simulink library "modbus_lib"  (Simulink 7.8)
settings: Solver=ode45  StartTime=0.0  StopTime=10.0  RelTol=1e-3
values from neighbouring files (symbols this model uses):
  relay_sets = xlsread('relay_settings_10272015.xlsx')    [relays_settings_init.m]
  Ts = 80e-6    (= 8e-05)    [global_parameters.m]    (also in scopeBuffer.m)
undefined symbols (not defined in the file or in its folder): angle_threshold, dF_threshold, DiscIntNeverNeededParam, dV_threshold, IOC, TOC, V, VRMSLL
libraries: simulink x24, powerlib_extras x20, powerlib x14, modbus_lib x6, simulink_extras x5, lib_Timer_Counter x4, rtio_generic_modbus x3, dspsigops x2
(part 2 of 2)

== system modbus_lib/CS Modified PLL/Controller ==
  note: Pierre Giroux, Gilbert Sybille
      | Power System Simulation Laboratory
      | IREQ, Hydro-Quebc
  note: Discrete PID Controller
  Error : Inport
  Discrete Derivative : simulink/Discrete/Discrete Derivative  gainval=1.0  ICPrevScaledInput=0.0  InputProcessing=Inherited  OutMin=[]  OutMax=[]  OutDataType=sfix(16)  OutScaling=2^-10  DoSatur=off
  Discrete-Time Integrator : DiscreteIntegrator  InitialCondition=Init  SampleTime=Ts  LimitOutput=on  UpperSaturationLimit=UpperLimit  LowerSaturationLimit=LowerLimit  ICPrevOutput=DiscIntNeverNeededParam  ICPrevScaledInput=DiscIntNeverNeededParam
  Kp4 : Gain  Gain=Kp  SaturateOnIntegerOverflow=on  OutDataTypeStr=Inherit: Same as input  ParamDataTypeStr=Inherit: Same as input
  Kp5 : Gain  Gain=Ki  SaturateOnIntegerOverflow=on  OutDataTypeStr=Inherit: Same as input  ParamDataTypeStr=Inherit: Same as input
  Kp6 : Gain  Gain=Kd  SaturateOnIntegerOverflow=on  OutDataTypeStr=Inherit: Same as input  ParamDataTypeStr=Inherit: Same as input
  Saturation2 : Saturate  UpperLimit=UpperLimit  LowerLimit=LowerLimit
  Sum6 : Sum  Inputs=+++  SaturateOnIntegerOverflow=on  InputSameDT=on  OutDataTypeStr=Inherit: Same as first input
  Zero-Order Hold : ZeroOrderHold  SampleTime=Ts
  Out : Outport  InitialOutput=0
  wires:
  Error/1 -> Kp4/1, Kp5/1, Kp6/1
  Sum6/1 -> Saturation2/1
  Kp5/1 -> Discrete-Time Integrator/1
  Kp6/1 -> Zero-Order Hold/1
  Kp4/1 -> Sum6/1
  Discrete-Time Integrator/1 -> Sum6/2
  Discrete Derivative/1 -> Sum6/3
  Saturation2/1 -> Out/1
  Zero-Order Hold/1 -> Discrete Derivative/1

== system modbus_lib/Gen_Synch/Freq_Comparator ==
  f_grid : Inport
  f_gen : Inport  Port=2
  Abs : Abs
  Compare To Constant2 : simulink/Logic and Bit Operations/Compare To Constant  relop=<=  const=0.2  OutDataTypeStr=uint8
  Fcn2 : Fcn  Expr=u(2)-u(1)
  Mux1 : Mux  Inputs=2
  Diff : Outport
  Locked : Outport  Port=2
  wires:
  Compare To Constant2/1 -> Locked/1
  f_grid/1 -> Mux1/1
  f_gen/1 -> Mux1/2
  Fcn2/1 -> Diff/1, Abs/1
  Mux1/1 -> Fcn2/1
  Abs/1 -> Compare To Constant2/1

== system modbus_lib/Gen_Synch/Freq_Controller ==
  f_diff : Inport
  Constant4 : Constant
  Gain1 : Gain  Gain=1/15  SampleTime=Ts
  Sum4 : Sum  Inputs=|-+  SampleTime=Ts
  F : Outport
  wires:
  Constant4/1 -> Sum4/2
  Sum4/1 -> F/1
  f_diff/1 -> Gain1/1
  Gain1/1 -> Sum4/1  "F"

== system modbus_lib/Gen_Synch/Phase_Comparator ==
  wt_grid : Inport
  wt_gen : Inport  Port=2
  Compare To Constant1 : simulink/Logic and Bit Operations/Compare To Constant  relop=<=  const=10  OutDataTypeStr=uint8
  Constant3 : Constant  Value=2*pi
  Fcn1 : Fcn  Expr=u(2)-u(1)  SampleTime=Ts
  Fcn3 : Fcn  Expr=abs(u(2)-u(1))  SampleTime=Ts
  Math Function : Math  Operator=mod  SampleTime=Ts  SaturateOnIntegerOverflow=on
  Mux3 : Mux  Inputs=2
  Radians to Degrees : simulink_extras/Transformations/Radians to Degrees
  Unwrap : dspsigops/Unwrap  tol=pi  InputProcessing=Columns as channels (frame based)  running=off
  Diff : Outport
  Locked : Outport  Port=2
  wires:
  Unwrap/1 -> Fcn3/1, Fcn1/1
  Math Function/1 -> Unwrap/1
  Compare To Constant1/1 -> Locked/1
  wt_gen/1 -> Mux3/2
  wt_grid/1 -> Mux3/1
  Fcn3/1 -> Radians to Degrees/1
  Mux3/1 -> Math Function/1
  Constant3/1 -> Math Function/2
  Radians to Degrees/1 -> Compare To Constant1/1
  Fcn1/1 -> Diff/1

== system modbus_lib/Gen_Synch/Phase_Controller ==
  wt_diff : Inport
  Constant5 : Constant
  Gain3 : Gain  Gain=1/(20*pi)  SampleTime=Ts
  Sum5 : Sum  Inputs=|-+  SampleTime=Ts
  F : Outport
  wires:
  Constant5/1 -> Sum5/2
  Sum5/1 -> F/1
  wt_diff/1 -> Gain3/1
  Gain3/1 -> Sum5/1  "F"

== system modbus_lib/Gen_Synch/RMS Calculator3 ==
  Vpeak : Inport
  Constant9 : Constant  Value=sqrt(3)
  Discrete  Mean value6 : powerlib_extras/Discrete Measurements/Discrete  Mean value  Freq=60  Vinit=0  Ts=Ts
  Product1 : Product  SampleTime=Ts  RndMeth=Zero
  Product3 : Product  SampleTime=Ts  RndMeth=Zero
  Signed Sqrt : Sqrt  SampleTime=Ts  SaturateOnIntegerOverflow=on
  VRMSLL : Outport
  wires:
  Discrete  Mean value6/1 -> Signed Sqrt/1
  Product3/1 -> Discrete  Mean value6/1
  Constant9/1 -> Product1/2
  Product1/1 -> Product3/2, Product3/1
  Vpeak/1 -> Product1/1
  Signed Sqrt/1 -> VRMSLL/1

== system modbus_lib/Gen_Synch/Subsystem ==
  V_grid : Inport
  V_gen : Inport  Port=2
  Discrete 1-phase PLL : powerlib_extras/Discrete  Control Blocks/Discrete 1-phase PLL  Fmin=45  Par_Init=[0 60]  ParK=[ 180 3200 1]  Ts=Ts  AGC=on
  Discrete 1-phase PLL1 : powerlib_extras/Discrete  Control Blocks/Discrete 1-phase PLL  Fmin=45  Par_Init=[0 60]  ParK=[ 180 3200 1]  Ts=Ts  AGC=on
  Gain : Gain  Gain=1/VRMSLL
  Gain1 : Gain  Gain=1/VRMSLL
  Terminator : Terminator
  Terminator1 : Terminator
  f_grid : Outport
  f_gen : Outport  Port=2
  wt_grid : Outport  Port=3
  wt_gen : Outport  Port=4
  wires:
  Discrete 1-phase PLL/2 -> wt_gen/1
  Discrete 1-phase PLL/1 -> f_gen/1
  Discrete 1-phase PLL1/2 -> wt_grid/1
  Discrete 1-phase PLL1/1 -> f_grid/1
  V_gen/1 -> Gain/1
  Gain/1 -> Discrete 1-phase PLL/1
  V_grid/1 -> Gain1/1
  Gain1/1 -> Discrete 1-phase PLL1/1
  Discrete 1-phase PLL/3 -> Terminator1/1
  Discrete 1-phase PLL1/3 -> Terminator/1

== system modbus_lib/Gen_Synch/Switch_Controller_Mode ==
  f_diff : Inport
  Op_Mode : Inport  Port=2
  Abs : Abs
  Compare To Constant : simulink/Logic and Bit Operations/Compare To Constant  relop=<=  const=0.2  OutDataTypeStr=boolean
  Compare To Constant1 : simulink/Logic and Bit Operations/Compare To Constant  relop===  const=1  OutDataTypeStr=boolean
  Compare To Constant5 : simulink/Logic and Bit Operations/Compare To Constant  relop===  const=2  OutDataTypeStr=boolean
  Constant6 : Constant
  Constant9 : Constant  Value=7500
  Logical Operator2 : Logic  AllPortsSameDT=off  OutDataTypeStr=boolean
  S-R Flip-Flop1 : simulink_extras/Flip Flops/S-R Flip-Flop  initial_condition=0
  Terminator : Terminator
  Terminator1 : Terminator
  Timer1 : lib_Timer_Counter/Timer
  Mode : Outport
  wires:
  Abs/1 -> Compare To Constant/1
  Logical Operator2/1 -> S-R Flip-Flop1/1
  Compare To Constant/1 -> Timer1/1
  Timer1/2 -> Logical Operator2/1
  Constant6/1 -> Timer1/3
  Constant9/1 -> Timer1/4
  Op_Mode/1 -> Compare To Constant5/1, Compare To Constant1/1
  Compare To Constant5/1 -> Timer1/2, S-R Flip-Flop1/2
  f_diff/1 -> Abs/1
  Compare To Constant1/1 -> Logical Operator2/2
  S-R Flip-Flop1/1 -> Mode/1
  S-R Flip-Flop1/2 -> Terminator/1
  Timer1/1 -> Terminator1/1

== system modbus_lib/Gen_Synch/Voltage_Comparator ==
  V_grid : Inport
  V_gen : Inport  Port=2
  Compare To Constant : simulink/Logic and Bit Operations/Compare To Constant  relop=<=  const=414  OutDataTypeStr=uint8
  Discrete Transfer Fcn : DiscreteTransferFcn  Numerator=[0.0004999]  Denominator=[1 -0.9995]  SampleTime=-1
  Fcn2 : Fcn  Expr=abs(u(2)-u(1))
  Mux1 : Mux  Inputs=2
  Diff : Outport
  Filt_Diff : Outport  Port=2
  Locked : Outport  Port=3
  wires:
  V_grid/1 -> Mux1/1
  V_gen/1 -> Mux1/2
  Discrete Transfer Fcn/1 -> Compare To Constant/1, Filt_Diff/1
  Compare To Constant/1 -> Locked/1
  Fcn2/1 -> Diff/1, Discrete Transfer Fcn/1
  Mux1/1 -> Fcn2/1

== system modbus_lib/Gen_Synch/Voltage_Controller ==
  V_gridRMS : Inport
  V_genRMS : Inport  Port=2
  Constant8 : Constant
  Divide : Product  Inputs=*/
  Sum1 : Sum  Inputs=|+-
  Sum3 : Sum  Inputs=|++
  V : Outport
  wires:
  Sum1/1 -> Divide/1
  Sum3/1 -> V/1  "V"
  Constant8/1 -> Sum3/2
  V_gridRMS/1 -> Sum1/1, Divide/2
  V_genRMS/1 -> Sum1/2
  Divide/1 -> Sum3/1

== system modbus_lib/Relay 25 - Sync Check - RS/Freq_Comparator ==
  note: This block compares the frequency at each of the circuit breaker terminals
      | * if the difference is less than threshold dF_threshold, then outputs 1
  f_grid : Inport
  f_gen : Inport  Port=2
  Abs : Abs
  Compare To Constant2 : simulink/Logic and Bit Operations/Compare To Constant  relop=<=  const=dF_threshold  OutDataTypeStr=uint8
  Fcn2 : Fcn  Expr=u(2)-u(1)
  Mux1 : Mux  Inputs=2
  Locked : Outport
  wires:
  Abs/1 -> Compare To Constant2/1
  Mux1/1 -> Fcn2/1
  Fcn2/1 -> Abs/1
  f_gen/1 -> Mux1/2
  f_grid/1 -> Mux1/1
  Compare To Constant2/1 -> Locked/1

== system modbus_lib/Relay 25 - Sync Check - RS/Phase_Comparator ==
  note: This block compares the angle (phase A only) at each of the circuit breaker terminals
      | * if the difference is less than threshold angle_threshold, then outputs 1
  wt_grid : Inport
  wt_gen : Inport  Port=2
  Compare To Constant1 : simulink/Logic and Bit Operations/Compare To Constant  relop=<=  const=angle_threshold  OutDataTypeStr=uint8
  Constant3 : Constant  Value=2*pi
  Fcn3 : Fcn  Expr=abs(u(2)-u(1))  SampleTime=Ts
  Math Function : Math  Operator=mod  SampleTime=Ts  SaturateOnIntegerOverflow=on
  Mux3 : Mux  Inputs=2
  Radians to Degrees : simulink_extras/Transformations/Radians to Degrees
  Unwrap : dspsigops/Unwrap  tol=pi  InputProcessing=Columns as channels (frame based)  running=off
  Locked : Outport
  wires:
  Radians to Degrees/1 -> Compare To Constant1/1  "R2D"
  Constant3/1 -> Math Function/2
  Mux3/1 -> Math Function/1
  Fcn3/1 -> Radians to Degrees/1  "diff"
  wt_grid/1 -> Mux3/1
  wt_gen/1 -> Mux3/2
  Compare To Constant1/1 -> Locked/1  "bool"
  Math Function/1 -> Unwrap/1
  Unwrap/1 -> Fcn3/1

== system modbus_lib/Relay 25 - Sync Check - RS/RMS ==
  s : Inport
  Discrete  Mean value6 : powerlib_extras/Discrete Measurements/Discrete  Mean value  Freq=60  Vinit=0  Ts=Ts
  Product3 : Product  RndMeth=Zero
  Signed Sqrt : Sqrt  SaturateOnIntegerOverflow=on
  S : Outport
  wires:
  s/1 -> Product3/1, Product3/2
  Product3/1 -> Discrete  Mean value6/1
  Discrete  Mean value6/1 -> Signed Sqrt/1
  Signed Sqrt/1 -> S/1

== system modbus_lib/Relay 25 - Sync Check - RS/Voltage_Comparator ==
  note: This block compares the frequency at each of the circuit breaker terminals
      | * if the difference is less than threshold dF_threshold, then outputs 1
  V_bus : Inport
  V_line : Inport  Port=2
  Fcn2 : Fcn  Expr=abs(u(2)-u(1))
  Mux1 : Mux  Inputs=2
  dV_threshold% of the nominal VRMSLL : simulink/Logic and Bit Operations/Compare To Constant  relop=<=  const=VRMSLL*dV_threshold  OutDataTypeStr=uint8
  Locked : Outport
  wires:
  Mux1/1 -> Fcn2/1
  Fcn2/1 -> dV_threshold% of the nominal VRMSLL/1  "diff"
  dV_threshold% of the nominal VRMSLL/1 -> Locked/1  "thshld"
  V_line/1 -> Mux1/2
  V_bus/1 -> Mux1/1

== system modbus_lib/Relay 25 - Sync Check - RS/set of 1ph PLLs ==
  V_bus : Inport
  V_line : Inport  Port=2
  Discrete 1-phase PLL : powerlib_extras/Discrete  Control Blocks/Discrete 1-phase PLL  Fmin=45  Par_Init=[0 60]  ParK=[ 180 3200 1]  Ts=Ts  AGC=on
  Discrete 1-phase PLL1 : powerlib_extras/Discrete  Control Blocks/Discrete 1-phase PLL  Fmin=45  Par_Init=[0 60]  ParK=[ 180 3200 1]  Ts=Ts  AGC=on
  Gain : Gain  Gain=1/VRMSLL
  Gain1 : Gain  Gain=1/VRMSLL
  Terminator : Terminator
  Terminator1 : Terminator
  f_bus : Outport
  f_line : Outport  Port=2
  wt_bus : Outport  Port=3
  wt_line : Outport  Port=4
  wires:
  Discrete 1-phase PLL1/3 -> Terminator1/1
  Discrete 1-phase PLL/3 -> Terminator/1
  Discrete 1-phase PLL/2 -> wt_line/1
  Discrete 1-phase PLL/1 -> f_line/1
  Discrete 1-phase PLL1/2 -> wt_bus/1
  Discrete 1-phase PLL1/1 -> f_bus/1
  V_line/1 -> Gain/1
  Gain/1 -> Discrete 1-phase PLL/1
  V_bus/1 -> Gain1/1
  Gain1/1 -> Discrete 1-phase PLL1/1

== system modbus_lib/SEL_787_Relay/PQ_Calculator ==
  Vabc : Inport
  Iabc : Inport  Port=2
  3-phase  Instantaneous  Active & Reactive Power : powerlib_extras/Measurements/3-phase  Instantaneous  Active & Reactive Power
  Demux : Demux  Outputs=2
  Discrete  Mean value2 : powerlib_extras/Discrete Measurements/Discrete  Mean value  Freq=60  Vinit=0  Ts=Ts
  P : Outport
  Q : Outport  Port=2
  wires:
  Demux/2 -> Q/1  "Q"
  Demux/1 -> P/1  "P"
  Iabc/1 -> 3-phase  Instantaneous  Active & Reactive Power/2
  Vabc/1 -> 3-phase  Instantaneous  Active & Reactive Power/1
  Discrete  Mean value2/1 -> Demux/1
  3-phase  Instantaneous  Active & Reactive Power/1 -> Discrete  Mean value2/1

== system modbus_lib/SEL_787_Relay/Phase_Calc ==
  note: Assumes Ib and Ic are shifted 120 degrees from Ia
      | For accurate phase measurements, could use a single-
      | phase PLL for each phase
  wt : Inport
  Add2 : Sum  Inputs=+-
  Add3 : Sum
  Constant5 : Constant  Value=120
  Constant6 : Constant  Value=120
  Constant7 : Constant  Value=2*pi
  Constant8 : Constant  Value=2*pi
  Math Function : Math  Operator=mod  SaturateOnIntegerOverflow=on
  Math Function1 : Math  Operator=mod  SaturateOnIntegerOverflow=on
  Phase a : Outport
  Phase b : Outport  Port=2
  Phase c : Outport  Port=3
  wires:
  Constant5/1 -> Add2/2
  Constant6/1 -> Add3/2
  wt/1 -> Add2/1, Phase a/1, Add3/1
  Constant7/1 -> Math Function/2
  Add2/1 -> Math Function/1
  Add3/1 -> Math Function1/1
  Constant8/1 -> Math Function1/2
  Math Function/1 -> Phase b/1
  Math Function1/1 -> Phase c/1

== system modbus_lib/SEL_787_Relay/Phase_Calc1 ==
  note: Assumes Ib and Ic are shifted 120 degrees from Ia
      | For accurate phase measurements, could use a single-
      | phase PLL for each phase
  wt : Inport
  Add2 : Sum  Inputs=+-
  Add3 : Sum
  Constant5 : Constant  Value=120
  Constant6 : Constant  Value=120
  Constant7 : Constant  Value=2*pi
  Constant8 : Constant  Value=2*pi
  Math Function : Math  Operator=mod  SaturateOnIntegerOverflow=on
  Math Function1 : Math  Operator=mod  SaturateOnIntegerOverflow=on
  Phase a : Outport
  Phase b : Outport  Port=2
  Phase c : Outport  Port=3
  wires:
  Math Function1/1 -> Phase c/1
  Math Function/1 -> Phase b/1
  Constant8/1 -> Math Function1/2
  Add3/1 -> Math Function1/1
  Add2/1 -> Math Function/1
  Constant7/1 -> Math Function/2
  wt/1 -> Add3/1, Phase a/1, Add2/1
  Constant6/1 -> Add3/2
  Constant5/1 -> Add2/2

== system modbus_lib/SEL_787_Relay/RMS_Calculator ==
  Signal : Inport
  Discrete  Mean value6 : powerlib_extras/Discrete Measurements/Discrete  Mean value  Freq=60  Vinit=0  Ts=Ts
  Product3 : Product  RndMeth=Zero
  Signed Sqrt : Sqrt  SaturateOnIntegerOverflow=on
  RMS_Signal : Outport
  wires:
  Signed Sqrt/1 -> RMS_Signal/1
  Discrete  Mean value6/1 -> Signed Sqrt/1
  Product3/1 -> Discrete  Mean value6/1
  Signal/1 -> Product3/2, Product3/1

== system modbus_lib/SEL_787_Relay/RMS_Calculator1 ==
  Signal : Inport
  Discrete  Mean value6 : powerlib_extras/Discrete Measurements/Discrete  Mean value  Freq=60  Vinit=0  Ts=Ts
  Product3 : Product  RndMeth=Zero
  Signed Sqrt : Sqrt  SaturateOnIntegerOverflow=on
  RMS_Signal : Outport
  wires:
  Signed Sqrt/1 -> RMS_Signal/1
  Discrete  Mean value6/1 -> Signed Sqrt/1
  Product3/1 -> Discrete  Mean value6/1
  Signal/1 -> Product3/2, Product3/1

== system modbus_lib/SEL_787_Relay/bitwise_faults ==
  note: Constant array has LSB on most left.
  S : Inport
  Bitwise Operator : simulink/Logic and Bit Operations/Bitwise Operator  logicop=OR  UseBitMask=off  NumInputPorts=7  BitMask=bin2dec('11011001')  BitMaskRealWorld=Stored Integer
  Data Type Conversion : DataTypeConversion  OutDataTypeStr=uint16
  Data Type Conversion1 : DataTypeConversion
  Demux : Demux  Outputs=7
  Shift Arithmetic : ArithShift  BitShiftNumber=1  BitShiftDirection=Left
  Shift Arithmetic1 : ArithShift  BitShiftNumber=2  BitShiftDirection=Left
  Shift Arithmetic2 : ArithShift  BitShiftNumber=3  BitShiftDirection=Left
  Shift Arithmetic3 : ArithShift  BitShiftNumber=4  BitShiftDirection=Left
  Shift Arithmetic4 : ArithShift  BitShiftNumber=5  BitShiftDirection=Left
  Shift Arithmetic5 : ArithShift  BitShiftNumber=6  BitShiftDirection=Left
  s : Outport
  wires:
  Data Type Conversion/1 -> Demux/1
  S/1 -> Data Type Conversion/1
  Bitwise Operator/1 -> Data Type Conversion1/1
  Data Type Conversion1/1 -> s/1
  Demux/1 -> Bitwise Operator/1
  Demux/2 -> Shift Arithmetic/1
  Demux/3 -> Shift Arithmetic1/1
  Demux/4 -> Shift Arithmetic2/1
  Demux/5 -> Shift Arithmetic3/1
  Demux/6 -> Shift Arithmetic4/1
  Demux/7 -> Shift Arithmetic5/1
  Shift Arithmetic/1 -> Bitwise Operator/2
  Shift Arithmetic1/1 -> Bitwise Operator/3
  Shift Arithmetic2/1 -> Bitwise Operator/4
  Shift Arithmetic3/1 -> Bitwise Operator/5
  Shift Arithmetic4/1 -> Bitwise Operator/6
  Shift Arithmetic5/1 -> Bitwise Operator/7

== system modbus_lib/SEL_787_Relay/pf bitwise ==
  note: Constant array has LSB on most left.
  S : Inport
  Bitwise Operator : simulink/Logic and Bit Operations/Bitwise Operator  logicop=OR  UseBitMask=off  NumInputPorts=2  BitMask=bin2dec('11011001')  BitMaskRealWorld=Stored Integer
  Data Type Conversion : DataTypeConversion  OutDataTypeStr=uint16
  Data Type Conversion1 : DataTypeConversion
  Demux : Demux  Outputs=2
  Shift Arithmetic : ArithShift  BitShiftNumber=1  BitShiftDirection=Left
  s : Outport
  wires:
  Shift Arithmetic/1 -> Bitwise Operator/2
  Demux/2 -> Shift Arithmetic/1
  Demux/1 -> Bitwise Operator/1
  Data Type Conversion1/1 -> s/1
  Bitwise Operator/1 -> Data Type Conversion1/1
  S/1 -> Data Type Conversion/1
  Data Type Conversion/1 -> Demux/1

== matlab function IEEE 1547 V&F/Over/Under Voltage/Frequency ==
  data: resetVoltage output double; Voltage_Trip_time output double; resetFreq output double; v input double; Frequency_Trip_time output double; va input double; vb input double; vc input double; freq input double; OF1 input double; OF2 input double; UF1 input double; UF2 input double; OV1 input double; OV2 input double; UV1 input double; UV2 input double; UV3 input double
function [  resetVoltage, Voltage_Trip_time, resetFreq, Frequency_Trip_time] = fcn(v, va, vb, vc, freq, OF1, OF2, UF1, UF2, OV1, OV2, UV1, UV2, UV3)

%This function implements time over/under voltage and over/under frequency.
%The clearing times are able to be set via the mask of the block.


resetA = 0;
resetB = 0;
resetC = 0;
resetFreq = 0;
timeA = inf;
timeB = inf;
timeC = inf;

if(0.45*v > va)
    timeA = UV1;
elseif((0.45*v <= va) && (va < 0.6*v))
    timeA = UV2;
elseif((0.6*v <= va) && (va < 0.88*v))
    timeA = UV3;
elseif((1.1*v < va) && (va < 1.2*v))
    timeA = OV1;
elseif(1.2*v < va)
    timeA = OV2;
else
    timeA = inf;
    resetA = 1;
end

if(0.45*v > vb)
    timeB = UV1;
elseif((0.45*v <= vb) && (vb < 0.6*v))
    timeB = UV2;
elseif((0.6*v <= vb) && (vb < 0.88*v))
    timeB = UV3;
elseif((1.1*v < vb) && (vb < 1.2*v))
    timeB = OV1;
elseif(1.2*v < vb)
    timeB = OV2;
else
    timeB = inf;
    resetB = 1;
end

if(0.45*v > vc)
    timeC = UV1;
elseif((0.45*v <= vc) && (vc < 0.6*v))
    timeC = UV2;
elseif((0.6*v <= vc) && (vc < 0.88*v))
    timeC = UV3;
elseif((1.1*v < vc) && (vc < 1.2*v))
    timeC = OV1;
elseif(1.2*v < vc)
    timeC = OV2;
else
    timeC = inf;
    resetC = 1;
end

if(freq <57)
    timeFreq = UF1;
elseif((57 <= freq) && (freq < 59.5))
    timeFreq = UF2;
elseif((60.5 <= freq) && (freq < 62))
    timeFreq = OF1;
elseif(freq >= 62)
    timeFreq = OF2;
else
    timeFreq = inf;
    resetFreq = 1;
end

time_vector = [timeA timeB timeC];
Voltage_Trip_time = min(time_vector);
Frequency_Trip_time = timeFreq;
resetVoltage = resetA & resetB & resetC;  %want to always reset timer time when all voltages are acceptable

== matlab function SEL_787_Relay/trip_out mng ==
  data: Ts input double; bool_R25 input double; op_mode_in input double; trip_out output double; trip_in input double; synch_check_time input double
function trip_out = opModeChk(Ts, bool_R25, op_mode_in, trip_in, synch_check_time)
%#codegen

persistent n25 prev_mode prev_trip_in
if isempty(prev_mode)
    n25 = 0; % time counter
    prev_mode = 0; % initially operating on logic
    prev_trip_in = 1; % initially close
end

trip_out = trip_in * bool_R25;

% the R25 logic will be active if the breaker has been opened, and a
% forced-to-close command is applied
if (prev_mode==2 || prev_trip_in==0) && (op_mode_in==1 || op_mode_in==0) && trip_in==1
    
    % time accumulation
    n25 = n25 * bool_R25;
    n25 = n25 + bool_R25 * Ts;
    if n25 > synch_check_time
        trip_out = 1;
        % reset history values
        prev_mode = op_mode_in;
        prev_trip_in = trip_in;
    else
        prev_mode = 2;
        prev_trip_in = 0;
        trip_out = 0;
    end
    
elseif op_mode_in==2
    prev_mode = 2;
    prev_trip_in = 0;
    trip_out = 0;
    n25 = 0;
else
    n25 = 0;
end

== matlab function bkr_control/MATLAB Function ==
  data: trip_in input double; logic_out output double; enable input double; status input double; time input double
function logic_out = fcn(trip_in, enable, status, time)
%#codegen

t_logic = 0.3; % time [sec] to activate logic
if enable == 1
    logic_out = status;
else
    if time > t_logic
        logic_out = trip_in;
    else
        logic_out = 1;
    end
end

== matlab function R50512759/Relays ==
  data: Ts input double; trip50 output double; Reset input double; Iinst input double; Irms input double; Vrms input double; IOC input double; trip51 output double; trip27 output double; TOC input double; VRMSLL input double; trip59 output double
function [trip50, trip51, trip27, trip59] = relays_50512759(Ts, Reset, Iinst, Irms, Vrms, IOC, TOC, VRMSLL)
%#codegen

% initialize or reset the trip signals
persistent R50 R51 R27 R59
if isempty(R51) || Reset
    R50=false;
    R51=false;
    R59=false;
    R27=false;
end

% latch for true signals
if ~(R50==true || R51==true)
    % calling external function
    r = relays50512759(Ts, Iinst, Irms, Vrms, IOC, TOC, VRMSLL);
    R50 = r.trip50;
    R51 = r.trip51;
    R27 = r.trip27;
    R59 = r.trip59;
end

trip50 = R50; % latched
trip51 = R51; % latched
trip27 = R27; % not latched
trip59 = R59; % not latched

== matlab function MATLAB Function ==
  data: trip_in input double; logic_out output double; enable input double; status input double; time input double
function logic_out = fcn(trip_in, enable, status, time)
%#codegen

t_logic = 0.3; % time [sec] to activate logic
if enable == 1
    logic_out = status;
else
    if time > t_logic
        logic_out = trip_in;
    else
        logic_out = 1;
    end
end

== matlab function Gen_Modbus_1MW/MATLAB Function ==
  data: Select_mb input double; P output double; P_mb input double; Q_mb input double; V_mb input double; F_mb input double; Mode_mb input double; Enable_mb input double; Q output double; V output double; F output double; Mode output double; Enable output double
function [P,Q,V,F,Mode,Enable] = genmb_1MW(Select_mb, P_mb, Q_mb, V_mb, F_mb, Mode_mb, Enable_mb)
%#codegen

if Select_mb == 1
    P = P_mb;
    Q = Q_mb;
    V = V_mb;
    F = F_mb;
    Mode = Mode_mb;
    Enable = Enable_mb;
else
    P = 0.8;
    Q = 0.2;
    V = 1;
    F = 1;
    Mode = 1;
    Enable = 1;
end

== matlab function Relay 25 - Sync Check - RS/deadbus fcn ==
  data: Vbus input double; y output double; Vline input double; VRMSLL input double
function y = fcn(Vbus, Vline, VRMSLL)
%#codegen
if isnan(Vbus)
    Vbus=0;
elseif isnan(Vline)
    Vline = 0;
end

% voltage threshold for deadbus
if VRMSLL > 400
    threshold = VRMSLL * 0.003; % @ 0.3%
else
    threshold = VRMSLL * 0.05; % @ 5%
end

% bounding open-circuit voltage at 120%
a = (Vbus>(VRMSLL*0.90)) && (Vbus<(VRMSLL*1.20)) && (Vline < threshold);
b = (Vline>(VRMSLL*0.90)) && (Vline<(VRMSLL*1.20)) && (Vbus < threshold);
c = (Vline < threshold) && (Vbus < threshold);
y = a||b||c;

== matlab function Gen_Modbus_4MW/MATLAB Function ==
  data: Select_mb input double; P output double; P_mb input double; Q_mb input double; V_mb input double; F_mb input double; Mode_mb input double; Enable_mb input double; Q output double; V output double; F output double; Mode output double; Enable output double; gen_cmds input double
function [P,Q,V,F,Mode,Enable] = genmb_4MW(Select_mb, P_mb, Q_mb, V_mb, F_mb, Mode_mb, Enable_mb, gen_cmds)
%#codegen

% gen_cmds mapping
if isempty(gen_cmds)
    Sync = 0;
    V_sync = 0;
    F_sync = 0;
    Mode_sync = 0;
else
    V_sync = gen_cmds(1);
    F_sync = gen_cmds(2);
    Mode_sync = gen_cmds(3);
    Sync = gen_cmds(4);
end

if Sync == 1
    VFM_select = 2;
else
    VFM_select = Select_mb;
end

if VFM_select == 1
    P = P_mb;
    Q = Q_mb;
    V = V_mb;
    F = F_mb;
    Mode = Mode_mb;
    Enable = Enable_mb;
elseif VFM_select == 2
    P = P_mb;
    Q = Q_mb;
    V = V_sync; % sync parameters
    F = F_sync;
    Mode = Mode_sync;
    Enable = Enable_mb;
else
    P = 0.8;
    Q = 0.2;
    V = 1;
    F = 1;
    Mode = 1;
    Enable = 1;
end

== matlab function BATT_MODBUS/MATLAB Function ==
  data: x input double; y output double
function y = fcn(x)
%#codegen

r=typecast(uint16(x),'int16');
y=double(r(1));

== matlab function BATT_MODBUS/MATLAB Function1 ==
  data: x input double; y output double
function y = fcn(x)
%#codegen

r=typecast(uint16(x),'int16');
y=double(r(1));

== matlab function trip_out mng ==
  data: Ts input double; bool_R25 input double; op_mode_in input double; trip_out output double; trip_in input double; synch_check_time input double
function trip_out = opModeChk(Ts, bool_R25, op_mode_in, trip_in, synch_check_time)
%#codegen

persistent n25 prev_mode prev_trip_in
if isempty(prev_mode)
    n25 = 0; % time counter
    prev_mode = 0; % initially operating on logic
    prev_trip_in = 1; % initially close
end

trip_out = trip_in * bool_R25;

% the R25 logic will be active if the breaker has been opened, and a
% forced-to-close command is applied
if (prev_mode==2 || prev_trip_in==0) && (op_mode_in==1 || op_mode_in==0) && trip_in==1
    
    % time accumulation
    n25 = n25 * bool_R25;
    n25 = n25 + bool_R25 * Ts;
    if n25 > synch_check_time
        trip_out = 1;
        % reset history values
        prev_mode = op_mode_in;
        prev_trip_in = trip_in;
    else
        prev_mode = 2;
        prev_trip_in = 0;
        trip_out = 0;
    end
    
elseif op_mode_in==2
    prev_mode = 2;
    prev_trip_in = 0;
    trip_out = 0;
    n25 = 0;
else
    n25 = 0;
end
